simulink model "heating_system"  (R2023b)
settings: Solver=VariableStepAuto  StartTime=0.0  StopTime=400.0  RelTol=1e-3
model workspace (MATLAB code in the model file):
  | % Contants
  | tau = 20;
  | Kp = 0.5;
  | sigma = 0.08;
  | alpha = 1E3;
  | beta = [1E-2; 1E-2];
  | delta_t = 0.1;
  | 
  | % Variables
  | a = -1 / tau;
  | b = Kp / tau;
  | W = 1 / sigma^2;
libraries: simulink x1
settings Model: Creator=eobregon  LastModifiedBy=eobregon

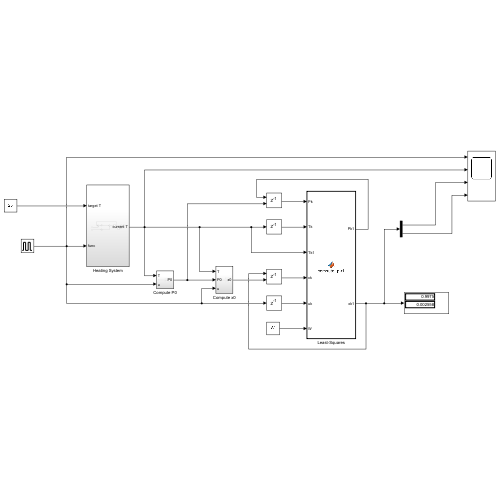
[thumbnail: Simulink's stored preview of the top-level diagram]
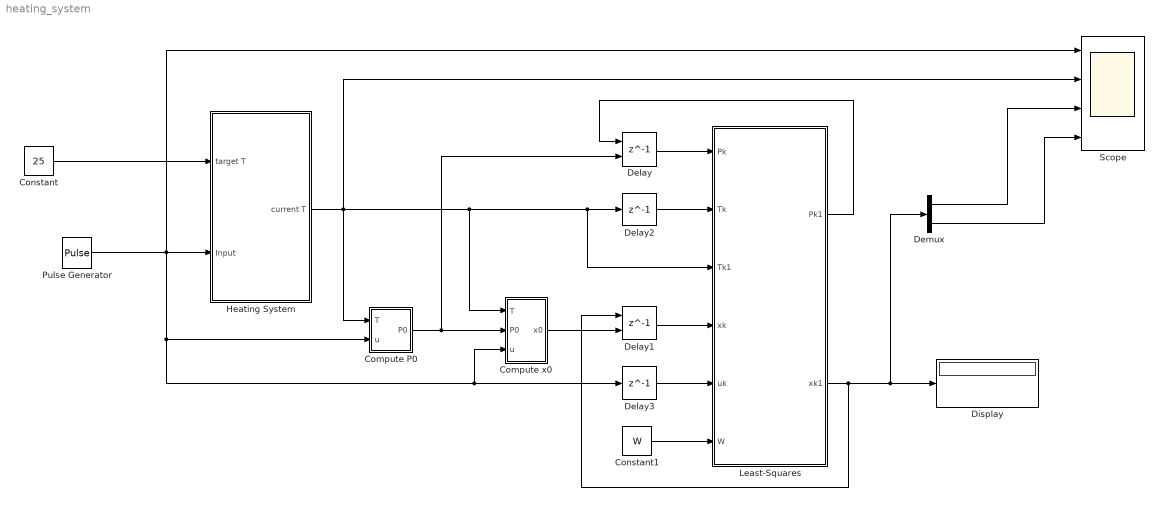
== system heating_system ==
  Compute P0 : Subsystem
  Compute x0 : Subsystem
  Constant : Constant  Value=25
  Constant1 : Constant  Value=W
  Delay : Delay  DelayLength=1  InitialConditionSource=Input port  InitialCondition=0  SampleTime=delta_t
      settings: InputPortMap=u0,p4
  Delay1 : Delay  DelayLength=1  InitialConditionSource=Input port  InitialCondition=0  SampleTime=delta_t
      settings: InputPortMap=u0,p4
  Delay2 : Delay  DelayLength=1  InitialCondition=0  SampleTime=delta_t
  Delay3 : Delay  DelayLength=1  InitialCondition=0  SampleTime=delta_t
  Demux : Demux  Outputs=2
  Display : Display
  Heating System : Subsystem
  Least-Squares : MATLAB Function  TreatAsAtomicUnit=on  SystemSampleTime=delta_t
  Pulse Generator : DiscretePulseGenerator  PulseType=Time based  Amplitude=100  Period=10  PulseWidth=50
  Scope : Scope  NumInputPorts=4
  wires:
  Constant/1 -> Heating System/1(target T)
  Heating System/1(current T) -> Scope/2, Compute P0/1(T), Compute x0/1(T), Least-Squares/3(Tk1), Delay2/1
  Pulse Generator/1 -> Delay3/1, Compute x0/3(u), Compute P0/2(u), Heating System/2(Input), Scope/1
  Delay/1 -> Least-Squares/1(Pk)
  Least-Squares/1(Pk1) -> Delay/1
  Compute P0/1(P0) -> Delay/2, Compute x0/2(P0)
  Delay1/1 -> Least-Squares/4(xk)
  Delay2/1 -> Least-Squares/2(Tk)
  Delay3/1 -> Least-Squares/5(uk)
  Compute x0/1(x0) -> Delay1/2
  Least-Squares/2(xk1) -> Display/1, Demux/1, Delay1/1
  Constant1/1 -> Least-Squares/6(W)
  Demux/1 -> Scope/3
  Demux/2 -> Scope/4

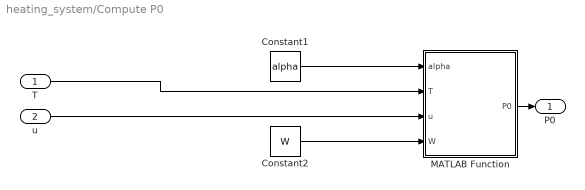
== system heating_system/Compute P0 ==
  T : Inport
  u : Inport  Port=2
  Constant1 : Constant  Value=alpha
  Constant2 : Constant  Value=W
  MATLAB Function : MATLAB Function  TreatAsAtomicUnit=on
  P0 : Outport
  wires:
  Constant1/1 -> MATLAB Function/1(alpha)
  MATLAB Function/1(P0) -> P0/1
  Constant2/1 -> MATLAB Function/4(W)
  T/1 -> MATLAB Function/2(T)
  u/1 -> MATLAB Function/3(u)

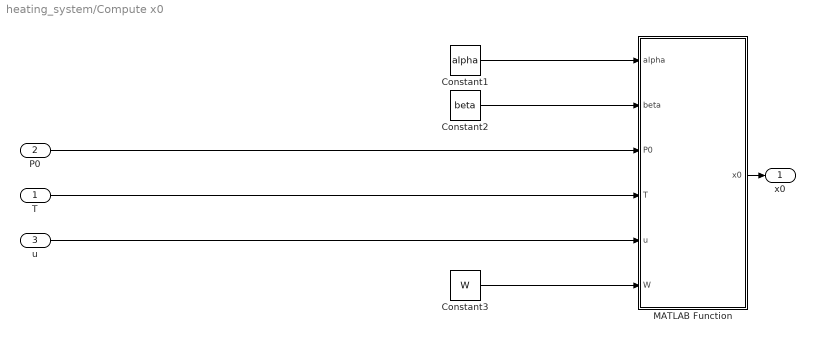
== system heating_system/Compute x0 ==
  T : Inport
  P0 : Inport  Port=2
  u : Inport  Port=3
  Constant1 : Constant  Value=alpha
  Constant2 : Constant  Value=beta
  Constant3 : Constant  Value=W
  MATLAB Function : MATLAB Function  TreatAsAtomicUnit=on
  x0 : Outport
  wires:
  Constant1/1 -> MATLAB Function/1(alpha)
  Constant3/1 -> MATLAB Function/6(W)
  Constant2/1 -> MATLAB Function/2(beta)
  MATLAB Function/1(x0) -> x0/1
  P0/1 -> MATLAB Function/3(P0)
  u/1 -> MATLAB Function/5(u)
  T/1 -> MATLAB Function/4(T)

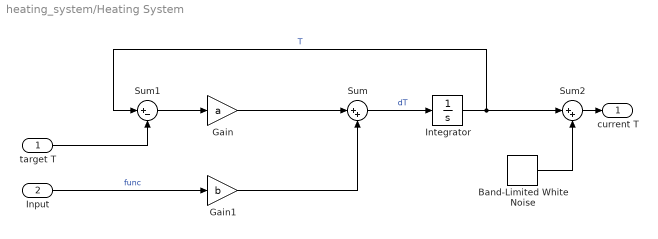
== system heating_system/Heating System ==
  target T : Inport
  Input : Inport  Port=2
  Band-Limited White Noise : simulink/Sources/Band-Limited White Noise  Cov=[0.05^2]  Ts=0.1  seed=[23341]
  Gain : Gain  Gain=a
  Gain1 : Gain  Gain=b
  Integrator : Integrator
  Sum : Sum  Inputs=|++
  Sum1 : Sum  Inputs=|+-
  Sum2 : Sum  Inputs=|++
  current T : Outport
  wires:
  Sum1/1 -> Gain/1
  Gain/1 -> Sum/1
  Sum/1 -> Integrator/1  "dT"
  target T/1 -> Sum1/2
  Integrator/1 -> Sum2/1, Sum1/1  "T"
  Band-Limited White Noise/1 -> Sum2/2
  Gain1/1 -> Sum/2
  Input/1 -> Gain1/1  "func"
  Sum2/1 -> current T/1

== matlab function heating_system/Least-Squares ==
  data: Pk input; Pk1 output; Tk input; Tk1 input; xk input; uk input; xk1 output; W input
function [Pk1, xk1] = compute_pk1(Pk, Tk, Tk1, xk, uk, W)
H = [Tk uk];
Ht = transpose(H);
I = eye(2);

K = Pk * Ht * inv(H * Pk * Ht + inv(W));
xk1 = xk + K * (Tk1 - H * xk);
Pk1 = (I - K * H) * Pk;

== matlab function heating_system/Compute P0/MATLAB Function ==
  data: alpha input; T input; u input; P0 output; W input
function P0 = compute_p0(alpha, T, u, W)
I = eye(2);
H = [T u];
Ht = transpose(H);

P0 = inv([1/alpha^2 * I + Ht * W * H]);

== matlab function heating_system/Compute x0/MATLAB Function ==
  data: alpha input; x0 output; beta input; P0 input; T input; u input; W input
function x0 = compute_x0(alpha, beta, P0, T, u, W)
H = [T u];
Ht = transpose(H);

x0 = P0 * (1 / alpha * beta + Ht * W * T);
